simulink library "HyEQ_Library_R2012a"  (R2017a)
settings: Solver=ode45  StartTime=0.0  StopTime=T  MaxStep=MaxStep  RelTol=RelTol  EnableMultiTasking=on
undefined symbols (not defined in the file): C, D, f, g, J, maxU, maxX, minU, rule, T, Tnmax, Tnmin, x0, x0ADC, x0NET
libraries: simulink x24
(part 3 of 3)

== matlab function HyEQ_Library_R2012a/Cyber Physical Systems/FSM/jump map g ==
  data: x input; xplus output; u input
function xplus = g(x, u)
%--------------------------------------------------------------------------
% Matlab M-file Project: HyEQ Toolbox @  Hybrid Systems Laboratory (HSL), 
% https://hybrid.soe.ucsc.edu/software
% http://hybridsimulator.wordpress.com/
%--------------------------------------------------------------------------
% Project: Simulation of a hybrid system Finite state machine (FSM)
% Description: Jump map
%--------------------------------------------------------------------------
%--------------------------------------------------------------------------
%   See also HYEQSOLVER, PLOTARC, PLOTARC3, PLOTFLOWS, PLOTHARC,
%   PLOTHARCCOLOR, PLOTHARCCOLOR3D, PLOTHYBRIDARC, PLOTJUMPS.
%   Copyright @ Hybrid Systems Laboratory (HSL),
%   Revision: 0.0.0.3 Date: 05/20/2015 3:42:00
%--------------------------------------------------------------------------
% jump map: xplus = g(x,u);

n = length(x); % size of the q state
qplus = zeros(n,1); % dynamics of the q state
% e.g., 
qplus(1) = 3-u(1);
qplus(2) = 3-u(2);

xplus = [qplus];

== matlab function HyEQ_Library_R2012a/Cyber Physical Systems/FSM/jump set D ==
  data: x input; v output; u input
function v  = D(x, u) 
%--------------------------------------------------------------------------
% Matlab M-file Project: HyEQ Toolbox @  Hybrid Systems Laboratory (HSL), 
% https://hybrid.soe.ucsc.edu/software
% http://hybridsimulator.wordpress.com/
%--------------------------------------------------------------------------
% Project: Simulation of a hybrid system Finite state machine (FSM)
% Description: Jump set
%--------------------------------------------------------------------------
%--------------------------------------------------------------------------
%   See also HYEQSOLVER, PLOTARC, PLOTARC3, PLOTFLOWS, PLOTHARC,
%   PLOTHARCCOLOR, PLOTHARCCOLOR3D, PLOTHYBRIDARC, PLOTJUMPS.
%   Copyright @ Hybrid Systems Laboratory (HSL),
%   Revision: 0.0.0.3 Date: 05/20/2015 3:42:00
%
% Check on jump conditions
% % E.g.,
% if (x(1) <= u(1)) && (x(2) <= 0)  % jump condition
%     v = 1;  % report jump
% else
%     v = 0;   % do not report jump
% end

n = length(x); % size of the q state
qplus = zeros(n,1); % dynamics of the q state
% e.g., 
qplus(1) = 3-u(1);
qplus(2) = 3-u(2);
if x(1)==qplus(1) && x(2)==qplus(2)
    v = 0; % do not report jump
else
    v = 1; % report jump
end

== matlab function HyEQ_Library_R2012a/Cyber Physical Systems/HSu/flow map f ==
  data: x input; xdot output; u input
function xdot = f(x, u)
%--------------------------------------------------------------------------
% Matlab M-file Project: HyEQ Toolbox @  Hybrid Systems Laboratory (HSL), 
% https://hybrid.soe.ucsc.edu/software
% http://hybridsimulator.wordpress.com/
%--------------------------------------------------------------------------
% Project: Simulation of a hybrid system (plant with constraints in the
% state and the input)
% Description: Flow map
%--------------------------------------------------------------------------
%--------------------------------------------------------------------------
%   See also HYEQSOLVER, PLOTARC, PLOTARC3, PLOTFLOWS, PLOTHARC,
%   PLOTHARCCOLOR, PLOTHARCCOLOR3D, PLOTHYBRIDARC, PLOTJUMPS.
%   Copyright @ Hybrid Systems Laboratory (HSL),
%   Revision: 0.0.0.3 Date: 05/20/2015 3:42:00
%--------------------------------------------------------------------------
% flow map: xdot=f(x,u);

x3 = x(3);
xdot = [sin(x3);cos(x3);u];

== matlab function HyEQ_Library_R2012a/Cyber Physical Systems/HSu/flow set C ==
  data: x input; v output; u input; minU parameter; maxU parameter; maxX parameter
function v  = C(x, u, minU, maxU, maxX) 
%--------------------------------------------------------------------------
% Matlab M-file Project: HyEQ Toolbox @  Hybrid Systems Laboratory (HSL), 
% https://hybrid.soe.ucsc.edu/software
% http://hybridsimulator.wordpress.com/
%--------------------------------------------------------------------------
% Project: Simulation of a hybrid system
% Description: Flow set
%--------------------------------------------------------------------------
%--------------------------------------------------------------------------
%   See also HYEQSOLVER, PLOTARC, PLOTARC3, PLOTFLOWS, PLOTHARC,
%   PLOTHARCCOLOR, PLOTHARCCOLOR3D, PLOTHYBRIDARC, PLOTJUMPS.
%   Copyright @ Hybrid Systems Laboratory (HSL),
%   Revision: 0.0.0.3 Date: 05/20/2015 3:42:00
%
% Check on flow conditions
% E.g.,
% if (x(1) >= u(1))  % flow condition
%     v = 1;  % report flow
% else
%     v = 0;   % do not report flow
% end

x1 = x(1);
x2 = x(2);


if u>=minU && u<=maxU && x1^2+x2^2<= maxX^2
    v = 1; % report flow
else
    v = 0; % do not report flow
end

== matlab function HyEQ_Library_R2012a/Cyber Physical Systems/HSu/jump map g ==
  data: x input; xplus output; u input
function xplus = g(x, u)
%--------------------------------------------------------------------------
% Matlab M-file Project: HyEQ Toolbox @  Hybrid Systems Laboratory (HSL), 
% https://hybrid.soe.ucsc.edu/software
% http://hybridsimulator.wordpress.com/
%--------------------------------------------------------------------------
% Project: Simulation of a hybrid system
% Description: Jump map
%--------------------------------------------------------------------------
%--------------------------------------------------------------------------
%   See also HYEQSOLVER, PLOTARC, PLOTARC3, PLOTFLOWS, PLOTHARC,
%   PLOTHARCCOLOR, PLOTHARCCOLOR3D, PLOTHYBRIDARC, PLOTJUMPS.
%   Copyright @ Hybrid Systems Laboratory (HSL),
%   Revision: 0.0.0.3 Date: 05/20/2015 3:42:00
%--------------------------------------------------------------------------
% jump map: xplus = g(x,u);

n = length(x);
xplus = zeros(n,1);

== matlab function HyEQ_Library_R2012a/Cyber Physical Systems/HSu/jump set D ==
  data: x input; v output; u input
function v  = D(x, u) 
%--------------------------------------------------------------------------
% Matlab M-file Project: HyEQ Toolbox @  Hybrid Systems Laboratory (HSL), 
% https://hybrid.soe.ucsc.edu/software
% http://hybridsimulator.wordpress.com/
%--------------------------------------------------------------------------
% Project: Simulation of a hybrid system
% Description: Jump set
%--------------------------------------------------------------------------
%--------------------------------------------------------------------------
%   See also HYEQSOLVER, PLOTARC, PLOTARC3, PLOTFLOWS, PLOTHARC,
%   PLOTHARCCOLOR, PLOTHARCCOLOR3D, PLOTHYBRIDARC, PLOTJUMPS.
%   Copyright @ Hybrid Systems Laboratory (HSL),
%   Revision: 0.0.0.3 Date: 05/20/2015 3:42:00
%
% Check on jump conditions
% % E.g.,
% if (x(1) <= u(1)) && (x(2) <= 0)  % jump condition
%     v = 1;  % report jump
% else
%     v = 0;   % do not report jump
% end

v = 0; % do not report jump

== matlab function HyEQ_Library_R2012a/Cyber Physical Systems/network/flow map f ==
  data: x input; xdot output; vs input
function xdot = f(x,vs)
%--------------------------------------------------------------------------
% Matlab M-file Project: HyEQ Toolbox @  Hybrid Systems Laboratory (HSL), 
% https://hybrid.soe.ucsc.edu/software
% http://hybridsimulator.wordpress.com/
%--------------------------------------------------------------------------
% Project: Simulation of a hybrid system Digital network (net) 
% Description: Flow map
%--------------------------------------------------------------------------
%--------------------------------------------------------------------------
%   See also HYEQSOLVER, PLOTARC, PLOTARC3, PLOTFLOWS, PLOTHARC,
%   PLOTHARCCOLOR, PLOTHARCCOLOR3D, PLOTHYBRIDARC, PLOTJUMPS.
%   Copyright @ Hybrid Systems Laboratory (HSL),
%   Revision: 0.0.0.3 Date: 05/20/2015 3:42:00

n = length(vs); % measured input size

msdot = zeros(n,1); % measured continuous dynamics
tau_sdot = -1; % Timer tau_s
xdot = [msdot;tau_sdot];

== matlab function HyEQ_Library_R2012a/Cyber Physical Systems/network/flow set C ==
  data: x input; v output; vs input; Tnmax parameter
function v  = C(x, vs, Tnmax) 
%--------------------------------------------------------------------------
% Matlab M-file Project: HyEQ Toolbox @  Hybrid Systems Laboratory (HSL), 
% https://hybrid.soe.ucsc.edu/software
% http://hybridsimulator.wordpress.com/
%--------------------------------------------------------------------------
% Project: Simulation of a hybrid system Digital network (net) 
% Description: Flow set
%--------------------------------------------------------------------------
%--------------------------------------------------------------------------
%   See also HYEQSOLVER, PLOTARC, PLOTARC3, PLOTFLOWS, PLOTHARC,
%   PLOTHARCCOLOR, PLOTHARCCOLOR3D, PLOTHYBRIDARC, PLOTJUMPS.
%   Copyright @ Hybrid Systems Laboratory (HSL),
%   Revision: 0.0.0.3 Date: 05/20/2015 3:42:00
%
% Check on flow conditions
% E.g.,
% if (x(1) >= u(1))  % flow condition
%     v = 1;  % report flow
% else
%     v = 0;   % do not report flow
% end

n = length(vs); % measured input size

tau_s = x(end); % timer state

if tau_s>=0 && tau_s<= Tnmax
    v = 1; % report flow
elseif tau_s> Tnmax
    v = 0; % do not report flow
else
    v = 0;
end

== matlab function HyEQ_Library_R2012a/Cyber Physical Systems/network/jump map g ==
  data: x input; xplus output; vs input; Tnmax parameter; Tnmin parameter
function xplus = g(x, vs, Tnmax, Tnmin)
%--------------------------------------------------------------------------
% Matlab M-file Project: HyEQ Toolbox @  Hybrid Systems Laboratory (HSL), 
% https://hybrid.soe.ucsc.edu/software
% http://hybridsimulator.wordpress.com/
%--------------------------------------------------------------------------
% Project: Simulation of a hybrid system Analog-to-Digital converter (ADC) 
% Description: Jump map
%--------------------------------------------------------------------------
%--------------------------------------------------------------------------
%   See also HYEQSOLVER, PLOTARC, PLOTARC3, PLOTFLOWS, PLOTHARC,
%   PLOTHARCCOLOR, PLOTHARCCOLOR3D, PLOTHYBRIDARC, PLOTJUMPS.
%   Copyright @ Hybrid Systems Laboratory (HSL),
%   Revision: 0.0.0.3 Date: 05/20/2015 3:42:00


n = length(vs); % measured input size

msplus = vs; % output = measured input
% The value tau_s is updated as a function of vs, e.g., 
tau_splus = mean(vs); % Timer tau_s
tau_splus = min(max(tau_splus,Tnmin),Tnmax);
xplus = [msplus;tau_splus];

== matlab function HyEQ_Library_R2012a/Cyber Physical Systems/network/jump set D ==
  data: x input; v output; vs input
function v  = D(x, vs) 
%--------------------------------------------------------------------------
% Matlab M-file Project: HyEQ Toolbox @  Hybrid Systems Laboratory (HSL), 
% https://hybrid.soe.ucsc.edu/software
% http://hybridsimulator.wordpress.com/
%--------------------------------------------------------------------------
% Project: Simulation of a hybrid system Analog-to-Digital converter (ADC) 
% Description: Jump set
%--------------------------------------------------------------------------
%--------------------------------------------------------------------------
%   See also HYEQSOLVER, PLOTARC, PLOTARC3, PLOTFLOWS, PLOTHARC,
%   PLOTHARCCOLOR, PLOTHARCCOLOR3D, PLOTHYBRIDARC, PLOTJUMPS.
%   Copyright @ Hybrid Systems Laboratory (HSL),
%   Revision: 0.0.0.3 Date: 05/20/2015 3:42:00
%
% Check on jump conditions
% % E.g.,
% if (x(1) <= u(1)) && (x(2) <= 0)  % jump condition
%     v = 1;  % report jump
% else
%     v = 0;   % do not report jump
% end

n = length(vs); % measured input size

tau_s = x(end); % timer state

if tau_s>=0
    v = 0; % do not report jump
elseif tau_s<= 0
    v = 1; % report jump
else
    v = 0;
end
